simulink model "IOT_Charger"  (R2024b)
settings: Solver=ode23tb  StartTime=0.0  StopTime=1  RelTol=1e-3  EnableMultiTasking=on
PreLoadFcn:
  | % Data of Solar Panel
  | %5000[W]/130[W]
  | % Total power generated by solar panel reaches 5[KW].
  | % each solar panel generates power 130[kW].
  | V = [0    40 80 120 160 180 200 217 240 260 280];
  | I = 5000/130*[0.68 0.675 0.67 0.665 0.660 0.655 0.640 0.6 0.48 0.28 0];
  | 
  | %subplot(211);plot(V,I);xlabel('Voltage[V]');ylabel('Current[a]')
  | %subplot(212);plot(V.*I);title('Power[W]')
  | 
  | % Sample Time[s]
  | Ts =5e-6;
  | 
  | 
  | %MPPT + PV Control
  | % PI control pamameter of Voltage control(Outer loop)
  | Kp_V = 50e-3;
  | Ki_V = 10;
  | 
  | % PI Control pamameter of Current control(Inner loop)
  | Kp_I = 25e-3;
  | Ki_I = 10;
  | 
  | % Utility Interconnection Control
  | % PI Control pamameter of Voltage control(Outer loop)
  | Kp_V2 = 0.01;
  | Ki_V2 = 25;
  | 
  | % PI control pamameter of Current control(Inner loop)
  | Kp_I2 = 0.01;
  | Ki_I2 = 25;
  | 
  | 
  | % Difference of voltege using in MPPT
  | dV = 0.5;
  | 
  | % Battery Control
  | % PI Control pamameter of Voltage control(Outer loop)
  | Kp_VB = 0.4;
  | Ki_VB = 2;
  | 
  | % PI control pamameter of Current control(Inner loop)
  | Kp_IB = 0.1;
  | Ki_IB = 0.5;
undefined symbols (not defined in the file): Ion, Lithium, sigbuilder_block
libraries: spsBreakerLib x120, spsSeriesRLCBranchLib x72, spsBatteryLib x43, spsIdealSwitchLib x29, spsVoltageMeasurementLib x25, spsMosfetLib x19, slpidlib x17, spsSeriesRLCLoadLib x12, spsPWMGeneratorDCDCLib x11, spsCurrentMeasurementLib x10, spsDiodeLib x6, spsPWMGenerator2LevelLib x5
(part 1 of 6)
Description:
  | Copyright 2008-2017 The MathWorks, Inc.
settings Model: SimulationMode=accelerator  Creator=MathWorks  LastModifiedBy=Jatay
settings SolverCC: ZeroCrossControl=DisableAll  ZeroCrossAlgorithm=Adaptive  AlgebraicLoopSolver=TrustRegion
settings DataIOCC: LimitDataPoints=on  SaveFormat=Array  SignalLoggingSaveFormat=ModelDataLogs  ReturnWorkspaceOutputs=off
settings OptimizationCC: ExpressionDepthLimit=2147483647  LifeSpan=inf
settings DebuggingCC: UnderspecifiedInitializationDetection=Classic  MergeDetectMultiDrivingBlocksExec=none  SolverPrmCheckMsg=warning  FcnCallInpInsideContextMsg=warning  UnconnectedInputMsg=warning  UnconnectedOutputMsg=warning  UnconnectedLineMsg=warning  AllowSymbolicDim=off  StateNameClashWarn=warning  SFUnexpectedBacktrackingDiag=warning  SFNoUnconditionalDefaultTransitionDiag=warning  SFExecutionAtInitializationDiag=none  ArithmeticOperatorsInVariantConditions=warning
settings HardwareCC: ProdBitPerPointer=32  ProdBitPerSizeT=32  ProdBitPerPtrDiffT=32  ProdLargestAtomicFloat=None  ProdIntDivRoundTo=Undefined  ProdEndianess=Unspecified  ProdWordSize=32  ProdHWDeviceType=32-bit Generic
settings ModelReferenceCC: EnableRefExpFcnMdlSchedulingChecks=on  PropagateSignalLabelsOutOfModel=off
settings SFSimCC: SimUseLocalCustomCode=off  SimParseCustomCode=off  CustomCodeUndefinedFunction=UseInterfaceOnly
settings RTWCC: RTWUseLocalCustomCode=off  GPUComputeCapability=3.5
settings CodeAppCC: StateflowObjectComments=on
settings GRTTargetCC: TargetLangStandard=C89/C90 (ANSI)  CombineOutputUpdateFcns=off  GRTInterface=on
settings ConfigComp: CovMetricSettings=dw  CovSaveCumulativeToWorkspaceVar=on  CovSaveSingleToWorkspaceVar=on  CovExternalEMLEnable=off  CovSFcnEnable=off
settings SimscapeCC: SimscapeNormalizeSystem=off

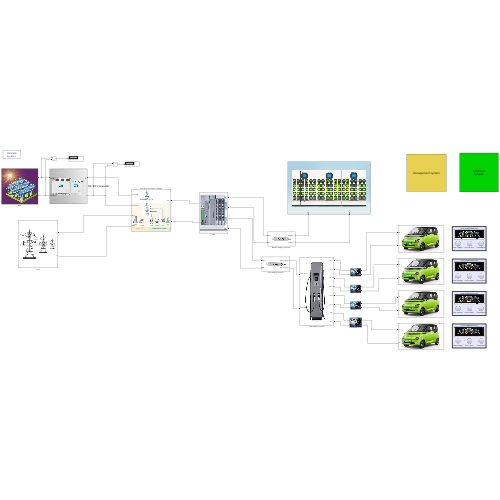
[thumbnail: Simulink's stored preview of the top-level diagram]
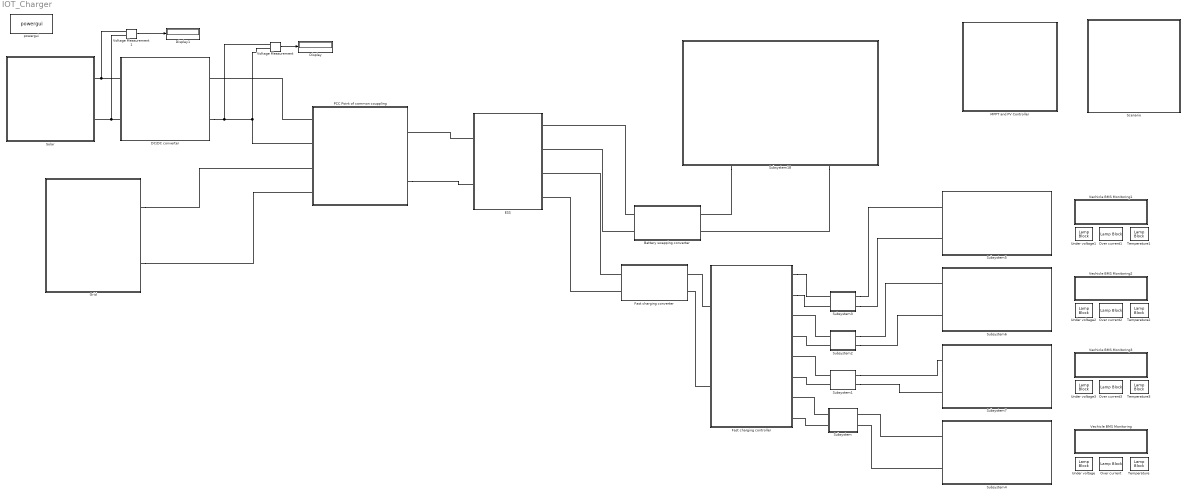
== system IOT_Charger ==
  Battery swapping converter : Subsystem
      mask Display: image('cc_converter.png');
  DC/DC converter : Subsystem
      mask Display: image('solar_controller.jpg');
  Display : Display
  Display1 : Display
  ESS : Subsystem
      mask Display: image('ess.jpeg');
  Fast charging controller : Subsystem
      mask Display: image('FC.jpeg');
  Fast charging converter : Subsystem
      mask Display: image('cc_converter.png');
  Grid : Subsystem
      mask Display: image('grid.png');
  MPPT and PV Controller : Subsystem
      mask Display: disp('Management system')
  Over current{,1..3} (4 alike) : LampBlock  LabelPosition=Hide
  PCC Point of common couppling : Subsystem
      mask Display: image('pcc.png');
  Scenario : Subsystem
      mask Display: disp('Additional\nScopes')
  Solar : Subsystem
      mask Display: image('Solar-Power-Plant-1024x536.jpg');
  Subsystem : Subsystem
      mask Display: image('plugin.jpeg');
  Subsystem1 : Subsystem
      mask Display: image('plugin.jpeg');
  Subsystem18 : Subsystem
      mask Display: image('swapping.webp');
  Subsystem2 : Subsystem
      mask Display: image('plugin.jpeg');
  Subsystem3 : Subsystem
      mask Display: image('plugin.jpeg');
  Subsystem4 : Subsystem
      mask Display: image('ev-1.jpeg');
  Subsystem5 : Subsystem
      mask Display: image('ev-1.jpeg');
  Subsystem6 : Subsystem
      mask Display: image('ev-1.jpeg');
  Subsystem7 : Subsystem
      mask Display: image('ev-1.jpeg');
  Temperature{,1..3} (4 alike) : LampBlock  LabelPosition=Hide
  Under voltage{,1..3} (4 alike) : LampBlock  LabelPosition=Hide
  Vechicle BMS Monitoring : Subsystem
      mask Display: image('Dash_board.jpeg');
  Vechicle BMS Monitoring1 : Subsystem
      mask Display: image('Dash_board.jpeg');
  Vechicle BMS Monitoring2 : Subsystem
      mask Display: image('Dash_board.jpeg');
  Vechicle BMS Monitoring3 : Subsystem
      mask Display: image('Dash_board.jpeg');
  Voltage Measurement : spsVoltageMeasurementLib/Voltage Measurement  PhasorSimulation=off  OutputType=Complex  PSBequivalent=0
  Voltage Measurement1 : spsVoltageMeasurementLib/Voltage Measurement  PhasorSimulation=off  OutputType=Complex  PSBequivalent=0
  powergui : spspowerguiLib/powergui  Priority=1  SimulationMode=Discrete  SampleTime=5e-6  frequency=60  Iterations=50  frequencyindice=0  Pbase=100e6  ErrMax=1e-4  UnitsV=kV  UnitsW=MW  buscounter=0  FunctionMessages=off  echomessages=off  EnableUseOfTLC=off  CurrentSourceSwitches=off  DisableSnubberDevices=off  DisableRonSwitches=off  DisableVfSwitches=off  DisplayEquations=off  AutomaticDiscreteSolvers=off  SolverType=Tustin  Interpol=off  ExternalGateDelay=off  methode=off  Ts=0  x0status=blocks  SPID=off  SwTol=0  HookPort=off  NonlinearTolerance=1e-4  nMaxIteration=100  ContinueOnMaxIteration=off  RestoreLinks=warning  ResistiveCurrentMeasurement=off  Frange=[0:2:500]  Ylog=off  Xlog=on  ShowGrid=off  save=off  variable=ZData  structure=0  ZoomFFT=off  StartTime=0.0  cycles=1  DisplayStyle=1  fundamental=60  FreqAxis=off  MaxFrequency=1000  frequencyindicesteady=1  RmsSteady=1  display=off
  wires:
  Voltage Measurement/1 -> Display/1
  Voltage Measurement1/1 -> Display1/1
  connections:
  DC/DC converter/LConn2 -- Voltage Measurement1/LConn2 -- Solar/RConn2
  DC/DC converter/LConn1 -- Voltage Measurement1/LConn1 -- Solar/RConn1
  PCC Point of common couppling/RConn2 -- ESS/LConn2
  ESS/LConn1 -- PCC Point of common couppling/RConn1
  PCC Point of common couppling/LConn1 -- DC/DC converter/RConn1
  DC/DC converter/RConn2 -- Voltage Measurement/LConn1 -- Voltage Measurement/LConn2 -- PCC Point of common couppling/LConn2
  Grid/RConn1 -- PCC Point of common couppling/LConn3
  Grid/RConn2 -- PCC Point of common couppling/LConn4
  Battery swapping converter/LConn1 -- ESS/RConn1
  Battery swapping converter/LConn2 -- ESS/RConn2
  Fast charging converter/LConn1 -- ESS/RConn3
  Fast charging converter/LConn2 -- ESS/RConn4
  Subsystem18/LConn1 -- Battery swapping converter/RConn1
  Subsystem18/LConn2 -- Battery swapping converter/RConn2
  Fast charging controller/LConn1 -- Fast charging converter/RConn2
  Fast charging controller/LConn2 -- Fast charging converter/RConn1
  Subsystem/LConn1 -- Fast charging controller/RConn2
  Subsystem/LConn2 -- Fast charging controller/RConn1
  Subsystem1/LConn2 -- Fast charging controller/RConn3
  Subsystem1/LConn1 -- Fast charging controller/RConn4
  Subsystem2/LConn2 -- Fast charging controller/RConn5
  Subsystem2/LConn1 -- Fast charging controller/RConn6
  Fast charging controller/RConn7 -- Subsystem3/LConn2
  Fast charging controller/RConn8 -- Subsystem3/LConn1
  Subsystem4/LConn1 -- Subsystem/RConn1
  Subsystem4/LConn2 -- Subsystem/RConn2
  Subsystem3/RConn1 -- Subsystem5/LConn1
  Subsystem3/RConn2 -- Subsystem5/LConn2
  Subsystem2/RConn1 -- Subsystem6/LConn1
  Subsystem2/RConn2 -- Subsystem6/LConn2
  Subsystem1/RConn1 -- Subsystem7/LConn1
  Subsystem1/RConn2 -- Subsystem7/LConn2

== system IOT_Charger/Battery swapping converter ==
  Current Measurement : spsCurrentMeasurementLib/Current Measurement  PhasorSimulation=off  OutputType=Complex  PSBequivalent=0
  Current Measurement1 : spsCurrentMeasurementLib/Current Measurement  PhasorSimulation=off  OutputType=Complex  PSBequivalent=0
  Current Measurement2 : spsCurrentMeasurementLib/Current Measurement  PhasorSimulation=off  OutputType=Complex  PSBequivalent=0
  Diode : spsDiodeLib/Diode  Ron=0.001  Lon=0  Vf=0.8  IC=0  UseSnubber=0  Rs=500  Cs=250e-9  Measurements=off
  Mosfet : spsMosfetLib/Mosfet  Ron=0.1  Lon=0  Rd=0.01  Vfd=0  IC=0  Rs=1e5  Cs=inf  Measurements=off
  Product : Product
  Pulse Generator : DiscretePulseGenerator  PulseType=Time based  Period=10  PulseWidth=5
  Scope2 : Scope  NumInputPorts=3
  Scope3 : Scope
  Scope4 : Scope
  Series RLC Branch : spsSeriesRLCBranchLib/Series RLC Branch  LConnTagsString=__new0  RConnTagsString=__new0  BranchType=L  Resistance=1  Inductance=1e-3  SetiL0=off  InitialCurrent=0  Capacitance=1e-6  Setx0=off  InitialVoltage=0  Measurements=None
  Series RLC Branch2 : spsSeriesRLCBranchLib/Series RLC Branch  LConnTagsString=__new0  RConnTagsString=__new0  BranchType=C  Resistance=1  Inductance=1e-3  SetiL0=off  InitialCurrent=0  Capacitance=1e-6  Setx0=off  InitialVoltage=0  Measurements=None
  Voltage Measurement : spsVoltageMeasurementLib/Voltage Measurement  PhasorSimulation=off  OutputType=Complex  PSBequivalent=0
  BB + : PMIOPort  Side=Left
  BB - : PMIOPort  Port=2  Side=Left
  Swapping + : PMIOPort  Port=3  Side=Right
  swapping - : PMIOPort  Port=4  Side=Right
  wires:
  Current Measurement/1 -> Scope2/1
  Voltage Measurement/1 -> Scope4/1, Product/1
  Current Measurement1/1 -> Scope2/3, Product/2
  Product/1 -> Scope3/1
  Current Measurement2/1 -> Scope2/2
  Pulse Generator/1 -> Mosfet/1
  connections:
  Series RLC Branch2/RConn1 -- BB -/RConn1 -- Series RLC Branch/RConn1 -- swapping -/RConn1 -- Voltage Measurement/LConn2
  Diode/LConn1 -- Current Measurement1/LConn1 -- Series RLC Branch2/LConn1
  BB +/RConn1 -- Current Measurement/LConn1
  Current Measurement1/RConn1 -- Swapping +/RConn1 -- Voltage Measurement/LConn1
  Mosfet/RConn1 -- Diode/RConn1 -- Current Measurement2/LConn1
  Current Measurement/RConn1 -- Mosfet/LConn1
  Current Measurement2/RConn1 -- Series RLC Branch/LConn1

== system IOT_Charger/DC//DC converter ==
  DC - DC Converter : Subsystem
  DC bus : Subsystem
  Display : Display
  Voltage Measurement : spsVoltageMeasurementLib/Voltage Measurement  PhasorSimulation=off  OutputType=Complex  PSBequivalent=0
  Voltage Measurement2 : spsVoltageMeasurementLib/Voltage Measurement  PhasorSimulation=off  OutputType=Complex  PSBequivalent=0
  solar + : PMIOPort  Side=Left
  solar - : PMIOPort  Port=2  Side=Left
  + : PMIOPort  Port=3  Side=Right
  - : PMIOPort  Port=4  Side=Right
  tag scope: solar_controller=global
  wires:
  Voltage Measurement2/1 -> [solar_controller]
  Voltage Measurement/1 -> Display/1
  connections:
  DC - DC Converter/RConn1 -- DC bus/LConn1
  solar +/RConn1 -- DC - DC Converter/LConn1 -- Voltage Measurement2/LConn1
  DC - DC Converter/LConn2 -- Voltage Measurement2/LConn2 -- solar -/RConn1
  DC - DC Converter/RConn2 -- DC bus/LConn2
  -/RConn1 -- DC bus/RConn2 -- Voltage Measurement/LConn2
  Voltage Measurement/LConn1 -- DC bus/RConn1 -- +/RConn1

== system IOT_Charger/ESS ==
  Battery : spsBatteryLib/Battery  BatType=Lithium-Ion  NomV=400  NomQ=40  SOC=80  Batt_Tr=30/10  PresetModel=on  MaxQ=40  MinV=300  FullV=465.5949  Dis_rate=17.3913  R=0.1  Normal_OP=36.1739  expZone="[432.1543      1.965217]"
  Battery Status : Scope  NumInputPorts=4
  Bus Selector : BusSelector  OutputSignals=SOC (%),Current (A),Voltage (V)
  Product1 : Product  RndMeth=Zero
  + : PMIOPort  Side=Left
  - : PMIOPort  Port=2  Side=Left
  BS + : PMIOPort  Port=3  Side=Right
  BS - : PMIOPort  Port=4  Side=Right
  FC + : PMIOPort  Port=5  Side=Right
  FC - : PMIOPort  Port=6  Side=Right
  tag scope: Power_Battery=global
  wires:
  Product1/1 -> [Power_Battery], Battery Status/4  "Power_Battery[W]"
  Battery/1 -> Bus Selector/1
  Bus Selector/3 -> Product1/2, Battery Status/3  "<Voltage (V)>"
  Bus Selector/2 -> Product1/1, Battery Status/2  "<Current (A)>"
  Bus Selector/1 -> Battery Status/1  "<SOC (%)>"
  connections:
  Battery/LConn2 -- -/RConn1 -- FC -/RConn1 -- BS -/RConn1
  Battery/LConn1 -- +/RConn1 -- FC +/RConn1 -- BS +/RConn1

== system IOT_Charger/Fast charging controller ==
  note: Solar
  Fast charging Switching controller : Subsystem
  Ideal Switch{,1..3} (4 alike) : spsIdealSwitchLib/Ideal Switch  Ron=0.001  Lon=0  IC=0  Rs=1e5  Cs=inf  Measurements=off
  solar panel - : PMIOPort  Side=Left
  solar panel + : PMIOPort  Port=2  Side=Left
  DC + : PMIOPort  Port=3  Side=Right
  DC - : PMIOPort  Port=4  Side=Right
  DC +1 : PMIOPort  Port=5  Side=Right
  DC +2 : PMIOPort  Port=6  Side=Right
  DC +3 : PMIOPort  Port=7  Side=Right
  DC +4 : PMIOPort  Port=8  Side=Right
  DC +5 : PMIOPort  Port=9  Side=Right
  DC +6 : PMIOPort  Port=10  Side=Right
  wires:
  [gg1] -> Ideal Switch3/1
  [gg2] -> Ideal Switch2/1
  [gg3] -> Ideal Switch1/1
  [gg4] -> Ideal Switch/1
  connections:
  Ideal Switch3/LConn1 -- Ideal Switch2/LConn1 -- Ideal Switch1/LConn1 -- Ideal Switch/LConn1 -- solar panel +/RConn1
  solar panel -/RConn1 -- DC +5/RConn1 -- DC +4/RConn1 -- DC +2/RConn1 -- DC -/RConn1
  Ideal Switch3/RConn1 -- DC +/RConn1
  Ideal Switch2/RConn1 -- DC +1/RConn1
  Ideal Switch1/RConn1 -- DC +3/RConn1
  Ideal Switch/RConn1 -- DC +6/RConn1

== system IOT_Charger/Fast charging converter ==
  Current Measurement : spsCurrentMeasurementLib/Current Measurement  PhasorSimulation=off  OutputType=Complex  PSBequivalent=0
  Current Measurement1 : spsCurrentMeasurementLib/Current Measurement  PhasorSimulation=off  OutputType=Complex  PSBequivalent=0
  Current Measurement2 : spsCurrentMeasurementLib/Current Measurement  PhasorSimulation=off  OutputType=Complex  PSBequivalent=0
  Diode : spsDiodeLib/Diode  Ron=0.001  Lon=0  Vf=0.8  IC=0  UseSnubber=0  Rs=500  Cs=250e-9  Measurements=off
  Mosfet : spsMosfetLib/Mosfet  Ron=0.1  Lon=0  Rd=0.01  Vfd=0  IC=0  Rs=1e5  Cs=inf  Measurements=off
  Product : Product
  Pulse Generator : DiscretePulseGenerator  PulseType=Time based  Period=10  PulseWidth=5
  Scope2 : Scope  NumInputPorts=3
  Scope3 : Scope
  Scope4 : Scope
  Series RLC Branch : spsSeriesRLCBranchLib/Series RLC Branch  LConnTagsString=__new0  RConnTagsString=__new0  BranchType=L  Resistance=1  Inductance=1e-3  SetiL0=off  InitialCurrent=0  Capacitance=1e-6  Setx0=off  InitialVoltage=0  Measurements=None
  Series RLC Branch2 : spsSeriesRLCBranchLib/Series RLC Branch  LConnTagsString=__new0  RConnTagsString=__new0  BranchType=C  Resistance=1  Inductance=1e-3  SetiL0=off  InitialCurrent=0  Capacitance=1e-6  Setx0=off  InitialVoltage=0  Measurements=None
  Voltage Measurement : spsVoltageMeasurementLib/Voltage Measurement  PhasorSimulation=off  OutputType=Complex  PSBequivalent=0
  BB + : PMIOPort  Side=Left
  BB - : PMIOPort  Port=2  Side=Left
  Fast charging + : PMIOPort  Port=3  Side=Right
  Fast charging - : PMIOPort  Port=4  Side=Right
  tag scope: FS=global
  wires:
  Current Measurement/1 -> Scope2/1
  Voltage Measurement/1 -> [FS], Scope4/1, Product/1
  Current Measurement1/1 -> Scope2/3, Product/2
  Product/1 -> Scope3/1
  Current Measurement2/1 -> Scope2/2
  Pulse Generator/1 -> Mosfet/1
  connections:
  Voltage Measurement/LConn2 -- Fast charging -/RConn1 -- Series RLC Branch2/RConn1 -- Series RLC Branch/RConn1 -- BB -/RConn1
  Diode/LConn1 -- Current Measurement1/LConn1 -- Series RLC Branch2/LConn1
  BB +/RConn1 -- Current Measurement/LConn1
  Current Measurement1/RConn1 -- Voltage Measurement/LConn1 -- Fast charging +/RConn1
  Mosfet/RConn1 -- Diode/RConn1 -- Current Measurement2/LConn1
  Current Measurement/RConn1 -- Mosfet/LConn1
  Current Measurement2/RConn1 -- Series RLC Branch/LConn1

== system IOT_Charger/Grid ==
  Display : Display
  Grid : spsThreePhaseSourceLib/Three-Phase Source  InternalConnection=Yg  VoltagePhases=off  Voltage=380  PhaseAngle=0  Voltage_phases=[25e3 25e3 25e3]/sqrt(3)  PhaseAngles_phases=[0 -120 +120]  Frequency=50  NonIdealSource=on  SpecifyImpedance=on  Resistance=0.8929  Inductance=16.58e-3  ShortCircuitLevel=100e6  BaseVoltage=380  XRratio=7  BusType=swing  Pref=10e3  Qref=0  Prefabc=[10e3, 10e3, 10e3]  Qrefabc=[0, 0, 0]  Qmin=-inf  Qmax=inf
  LOAD1 : spsThreePhaseSeriesRLCLoadLib/Three-Phase Series RLC Load  LConnTagsString=A|B|C  Configuration=Y (grounded)  NominalVoltage=380  Vabc=[1e3 1e3 1e3]  Vabcp=[1e3 1e3 1e3]  NominalFrequency=50  UnbalancedPower=off  ActivePower=1e3  InductivePower=0  CapacitivePower=0  Pabc=[10e3 9e3 11e3]  QLabc=[100 90 110]  QCabc=[100 90 110]  Pabcp=[10e3 9e3 11e3]  QLabcp=[100 90 110]  QCabcp=[100 90 110]  Measurements=None  LoadType=constant Z
  Measurement : spsThreePhaseVIMeasurementLib/Three-Phase V-I Measurement  VoltageMeasurement=phase-to-phase  SetLabelV=on  LabelV=Vabc_grid  Vpu=off  VpuLL=off  CurrentMeasurement=yes  SetLabelI=on  LabelI=Iabc_grid  Ipu=off  Pbase=100e6  Vbase=500e3  OutputType=Complex  PhasorSimulation=off  PSBequivalent=0
  Mux : Mux  Inputs=2
  Repeating Sequence Stair : simulink/Sources/Repeating Sequence Stair  OutValues=[0 0 1 1 0].'  tsamp=0.1  OutMin=[]  OutMax=[]  OutDataTypeStr=double  OutputDataTypeScalingMode=double  OutDataType=fixdt(0,8)  ConRadixGroup=Best Precision: Vector-wise  OutScaling=2^-12
  Scope : Scope
  Scope1 : Scope
  Scope2 : Scope  NumInputPorts=2
  V2G & G2V results : Scope  NumInputPorts=3
  Voltage Measurement : spsVoltageMeasurementLib/Voltage Measurement  PhasorSimulation=off  OutputType=Complex  PSBequivalent=0
  Wall charger Connection Box : Subsystem
  + : PMIOPort  Side=Right
  +1 : PMIOPort  Port=2  Side=Right
  tag scope: Control=global
  wires:
  [Control] -> Wall charger Connection Box/1(Control)
  Mux/1 -> V2G & G2V results/3
  [Vabc_grid] -> V2G & G2V results/1
  [Vabc_inv] -> V2G & G2V results/2
  Repeating Sequence Stair/1 -> [Control], Scope1/1
  [Vabc_inv] -> Mux/2
  [Iabc_out] -> Scope2/2
  [Iabc_inv] -> Scope/1
  [Vabc_out] -> Scope2/1
  Voltage Measurement/1 -> Display/1
  [Vabc_grid] -> Mux/1
  connections:
  Wall charger Connection Box/RConn2 -- Voltage Measurement/LConn2 -- +1/RConn1
  Grid/RConn1 -- Measurement/LConn1
  Grid/RConn3 -- Measurement/LConn3
  Wall charger Connection Box/RConn1 -- Voltage Measurement/LConn1 -- +/RConn1
  Grid/RConn2 -- Measurement/LConn2
  LOAD1/LConn3 -- Measurement/RConn3 -- Wall charger Connection Box/LConn3
  Measurement/RConn2 -- LOAD1/LConn2 -- Wall charger Connection Box/LConn2
  Measurement/RConn1 -- LOAD1/LConn1 -- Wall charger Connection Box/LConn1

== system IOT_Charger/MPPT and PV Controller ==
  Battery controller : Subsystem
  Inverter controller : Subsystem
  MMPT Controller : Subsystem
  Solar controller : Subsystem
  Swapping battery controller : Subsystem

== system IOT_Charger/PCC Point of common couppling ==
  note: ESS
  note: Grid
  note: Solar
  Display : Display
  Display1 : Display
  Display2 : Display
  Voltage Measurement : spsVoltageMeasurementLib/Voltage Measurement  PhasorSimulation=off  OutputType=Complex  PSBequivalent=0
  Voltage Measurement1 : spsVoltageMeasurementLib/Voltage Measurement  PhasorSimulation=off  OutputType=Complex  PSBequivalent=0
  Voltage Measurement2 : spsVoltageMeasurementLib/Voltage Measurement  PhasorSimulation=off  OutputType=Complex  PSBequivalent=0
  DC + : PMIOPort  Side=Right
  solar panel + : PMIOPort  Port=2  Side=Left
  solar panel - : PMIOPort  Port=3  Side=Left
  DC - : PMIOPort  Port=4  Side=Right
  Grid + : PMIOPort  Port=5  Side=Left
  Grid - : PMIOPort  Port=6  Side=Left
  wires:
  Voltage Measurement/1 -> Display/1
  Voltage Measurement1/1 -> Display1/1
  Voltage Measurement2/1 -> Display2/1
  connections:
  DC +/RConn1 -- Voltage Measurement2/LConn1 -- Voltage Measurement1/LConn1 -- Grid +/RConn1 -- Voltage Measurement/LConn1 -- solar panel +/RConn1
  solar panel -/RConn1 -- Voltage Measurement/LConn2 -- Grid -/RConn1 -- Voltage Measurement1/LConn2 -- Voltage Measurement2/LConn2 -- DC -/RConn1

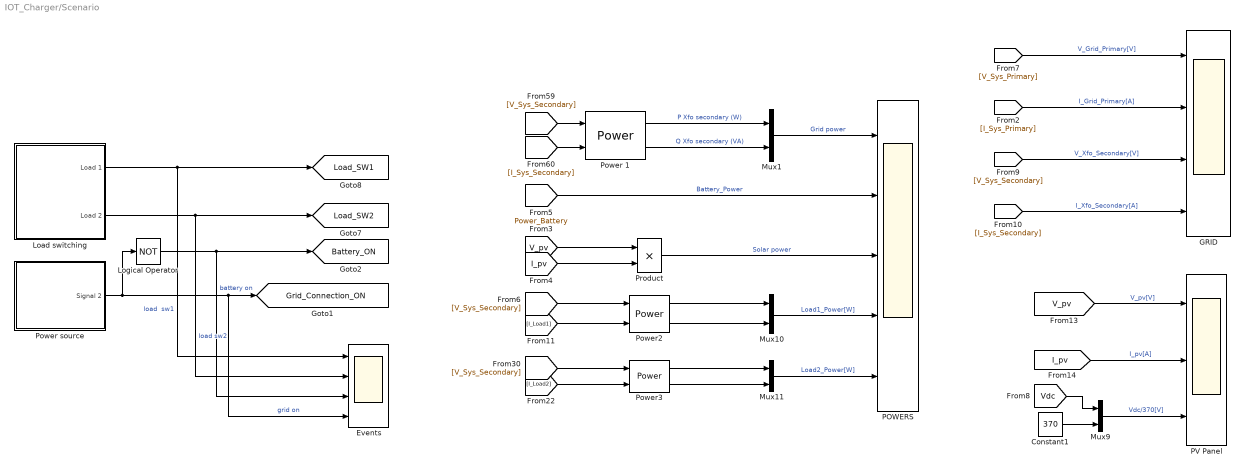
== system IOT_Charger/Scenario ==
  Constant1 : Constant  Value=370
  Events : Scope  NumInputPorts=4
  GRID : Scope  NumInputPorts=4
  Load switching : Subsystem  Tag=STV Subsys  LoadFcn=sigbuilder_block('load');  StartFcn=sigbuilder_block('start');  StopFcn=sigbuilder_block('stop');  ClipboardFcn=sigbuilder_block('clipboard');  mask(Sigbuilder block){tuvar=[0:10]}
      mask help: Simulink:masks:SigbuilderBlock_MD
      mask init:
      | if ~strcmp(get_param(bdroot(gcbh),'SimulationStatus'),'stopped') tuvar = sigbuilder_block('maskInit'); end
      settings: CopyFcn=sigbuilder_block('copy');  DeleteFcn=sigbuilder_block('delete');  ModelCloseFcn=sigbuilder_block('modelClose');  PreSaveFcn=sigbuilder_block('preSave');  PauseFcn=sigbuilder_block('pause');  ContinueFcn=sigbuilder_block('continue');  NameChangeFcn=sigbuilder_block('namechange');  OpenFcn=sigbuilder_block('open',[57 105.75 1180.5 663.75 ]);  CloseFcn=sigbuilder_block('close');
      mask Display: plot(0, 0, 100, 100,[2, 2, 32, 32, 2], [68, 8, 8, 68, 68],[32, 2], [38, 38], [32, 19, 2],[53, 60, 44], [32, 17, 17, 2],[16, 16, 31, 31]);txt = getActiveGroup(gcbh);text(2, 100, txt,'verticalAlignment', 'top');
  Logical Operator : Logic  Operator=NOT  AllPortsSameDT=off  OutDataTypeStr=boolean
  Mux{1,9..11} (4 alike) : Mux  Inputs=2
  POWERS : Scope  NumInputPorts=5
  PV Panel : Scope  NumInputPorts=3
  Power 1 : spsPowerLib/Power  Freq=60  Vinit=[1, 0]  Iinit=[1, 0]  Ts=0
  Power source : Subsystem  Tag=STV Subsys  LoadFcn=sigbuilder_block('load');  StartFcn=sigbuilder_block('start');  StopFcn=sigbuilder_block('stop');  ClipboardFcn=sigbuilder_block('clipboard');  mask(Sigbuilder block){tuvar=[0:10]}
      mask help: Simulink:masks:SigbuilderBlock_MD
      mask init:
      | if ~strcmp(get_param(bdroot(gcbh),'SimulationStatus'),'stopped') tuvar = sigbuilder_block('maskInit'); end
      settings: CopyFcn=sigbuilder_block('copy');  DeleteFcn=sigbuilder_block('delete');  ModelCloseFcn=sigbuilder_block('modelClose');  PreSaveFcn=sigbuilder_block('preSave');  PauseFcn=sigbuilder_block('pause');  ContinueFcn=sigbuilder_block('continue');  NameChangeFcn=sigbuilder_block('namechange');  OpenFcn=sigbuilder_block('open',[436.966 199.241 549.931 400.345 ]);  CloseFcn=sigbuilder_block('close');
      mask Display: plot(0, 0, 100, 100,[2, 2, 32, 32, 2], [68, 8, 8, 68, 68],[32, 2], [38, 38], [32, 19, 2],[53, 60, 44], [32, 17, 17, 2],[16, 16, 31, 31]);txt = getActiveGroup(gcbh);text(2, 100, txt,'verticalAlignment', 'top');
  Power2 : spsPowerLib/Power  Freq=60  Vinit=[1, 0]  Iinit=[1, 0]  Ts=0
  Power3 : spsPowerLib/Power  Freq=60  Vinit=[1, 0]  Iinit=[1, 0]  Ts=0
  Product : Product  RndMeth=Zero
  tag scope: Battery_ON=global, Grid_Connection_ON=global, Load_SW1=global, Load_SW2=global
  wires:
  Load switching/2(Load 2) -> [Load_SW2], Events/2  "load sw2"
  Logical Operator/1 -> Events/3, [Battery_ON]  "battery on"
  Power source/1(Signal 2) -> Events/4, [Grid_Connection_ON], Logical Operator/1  "grid on"
  Load switching/1(Load 1) -> [Load_SW1], Events/1  "load  sw1"
  [Vdc] -> Mux9/1
  Constant1/1 -> Mux9/2
  Mux9/1 -> PV Panel/3  "Vdc/370[V]"
  [V_Sys_Primary] -> GRID/1  "V_Grid_Primary[V]"
  [I_Sys_Primary] -> GRID/2  "I_Grid_Primary[A]"
  [V_Sys_Secondary] -> GRID/3  "V_Xfo_Secondary[V]"
  [I_Sys_Secondary] -> GRID/4  "I_Xfo_Secondary[A]"
  [V_pv] -> PV Panel/1  "V_pv[V]"
  [I_pv] -> PV Panel/2  "I_pv[A]"
  [V_pv] -> Product/1
  [I_pv] -> Product/2
  Product/1 -> POWERS/3  "Solar power"
  [Power_Battery] -> POWERS/2  "Battery_Power"
  [V_Sys_Secondary] -> Power 1/1
  [I_Sys_Secondary] -> Power 1/2
  [V_Sys_Secondary] -> Power2/1
  [I_Load1] -> Power2/2
  Mux10/1 -> POWERS/4  "Load1_Power[W]"
  [V_Sys_Secondary] -> Power3/1
  [I_Load2] -> Power3/2
  Mux11/1 -> POWERS/5  "Load2_Power[W]"
  Power2/1 -> Mux10/1
  Power2/2 -> Mux10/2
  Power3/1 -> Mux11/1
  Power3/2 -> Mux11/2
  Mux1/1 -> POWERS/1  "Grid power"
  Power 1/1 -> Mux1/1  "P Xfo secondary (W)"
  Power 1/2 -> Mux1/2  "Q Xfo secondary (VA)"

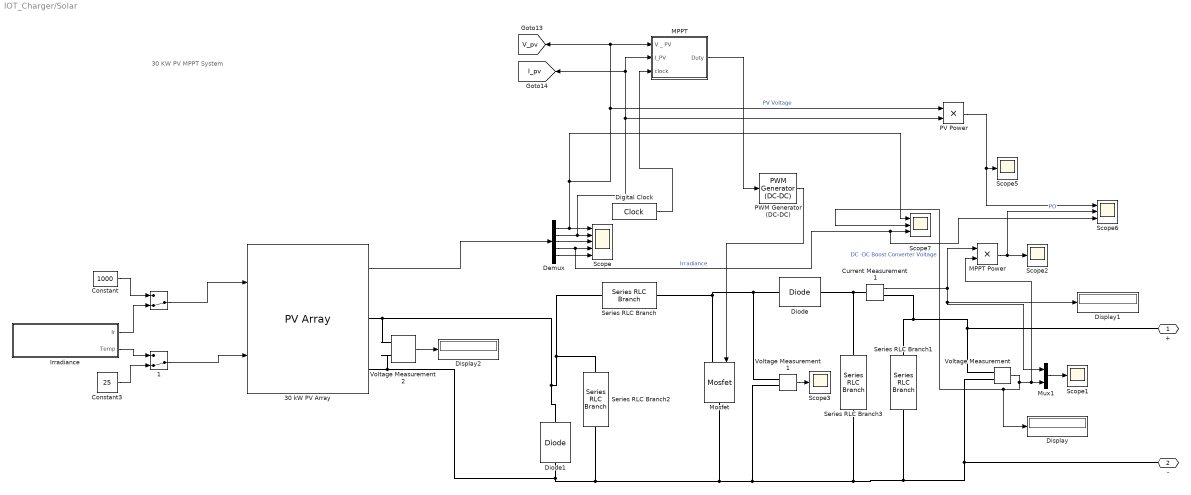
== system IOT_Charger/Solar ==
  note: 30 KW PV MPPT System
  "      " : ManualSwitch  CurrentSetting=0
  "      1" : ManualSwitch  CurrentSetting=0
  30 kW PV Array : spsPVArrayLib/PV Array  Npar=15  Nser=10  PlotType=array @ 1000 W/m2 & specified temperatures  S_vec="[ 1000  500  100 ]"  Temp_C_vec="[ 45 25  ]"  ModuleName=User-defined  PlotWhenSelected=off  Pm=213.15  Ncell=60  Voc=48  Isc=7.84  Vm=29  Im=7.35  beta_Voc_pc=-0.36099  alpha_Isc_pc=0.102  beta_Voc=-0.17328  alpha_Isc=0.0079968  IL=8.2285  I0=2.9956e-10  nI=1.2955  Rsh=7353.5939  Rs=2.0228  RobustModel=off  RobustCellTemperature=25  BAL=on  Tc=1e-6  Tfilter=5e-5
  Constant : Constant  Value=1000
  Constant3 : Constant  Value=25
  Current Measurement1 : spsCurrentMeasurementLib/Current Measurement  PhasorSimulation=off  OutputType=Complex  PSBequivalent=0
  Demux : Demux  Outputs=5
  Digital Clock : DigitalClock  SampleTime=0.001
  Diode : spsDiodeLib/Diode  Ron=0.5  Lon=0  Vf=0.7  IC=0  UseSnubber=0  Rs=1e5  Cs=250e-9  Measurements=off
  Diode1 : spsDiodeLib/Diode  Ron=0.5  Lon=0  Vf=0.7  IC=0  UseSnubber=0  Rs=1e5  Cs=250e-9  Measurements=off
  Display : Display
  Display1 : Display
  Display2 : Display
  "Irradiance " : Subsystem  Tag=STV Subsys  LoadFcn=sigbuilder_block('load');  StartFcn=sigbuilder_block('start');  StopFcn=sigbuilder_block('stop');  ClipboardFcn=sigbuilder_block('clipboard');  mask(Sigbuilder block){tuvar=[0:10]}
      mask help: Sigbuilder GUI
      mask init:
      | if ~strcmp(get_param(bdroot(gcbh),'SimulationStatus'),'stopped') tuvar = sigbuilder_block('maskInit'); end
      settings: CopyFcn=sigbuilder_block('copy');  DeleteFcn=sigbuilder_block('delete');  ModelCloseFcn=sigbuilder_block('modelClose');  PreSaveFcn=sigbuilder_block('preSave');  PauseFcn=sigbuilder_block('pause')  ContinueFcn=sigbuilder_block('continue')  NameChangeFcn=sigbuilder_block('namechange');  OpenFcn=sigbuilder_block('open',[5.4 30 1141.2 507.6 ]);  CloseFcn=sigbuilder_block('close');
      mask Display: plot(0, 0, 100, 100,[2, 2, 32, 32, 2], [68, 8, 8, 68, 68],[32, 2], [38, 38], [32, 19, 2],[53, 60, 44], [32, 17, 17, 2],[16, 16, 31, 31]);txt = getActiveGroup(gcbh);text(2, 100, txt,'verticalAlignment', 'top');
  MPPT : Subsystem
  MPPT Power : Product
  Mosfet : spsMosfetLib/Mosfet  Ron=0.1  Lon=0  Rd=0.01  Vfd=0.7  IC=0  Rs=1e5  Cs=inf  Measurements=off
  Mux1 : Mux  Inputs=2
  PV Power : Product
  PWM Generator (DC-DC) : spsPWMGeneratorDCDCLib/PWM Generator (DC-DC)  Fsw=1500  Ts=0
  Scope : Scope  NumInputPorts=5
  Scope{1..3,5} (4 alike) : Scope
  Scope6 : Scope  NumInputPorts=3
  Scope7 : Scope  NumInputPorts=3
  Series RLC Branch : spsSeriesRLCBranchLib/Series RLC Branch  LConnTagsString=__new0  RConnTagsString=__new0  BranchType=L  Resistance=0.001  Inductance=0.4e-1  SetiL0=off  InitialCurrent=0  Capacitance=1e-6  Setx0=off  InitialVoltage=0  Measurements=None
  Series RLC Branch1 : spsSeriesRLCBranchLib/Series RLC Branch  LConnTagsString=__new0  RConnTagsString=__new0  BranchType=R  Resistance=11  Inductance=0.1  SetiL0=off  InitialCurrent=0  Capacitance=100e-6  Setx0=off  InitialVoltage=0  Measurements=None
  Series RLC Branch2 : spsSeriesRLCBranchLib/Series RLC Branch  LConnTagsString=__new0  RConnTagsString=__new0  BranchType=C  Resistance=6  Inductance=0.1  SetiL0=off  InitialCurrent=0  Capacitance=700e-5  Setx0=off  InitialVoltage=0  Measurements=None
  Series RLC Branch3 : spsSeriesRLCBranchLib/Series RLC Branch  LConnTagsString=__new0  RConnTagsString=__new0  BranchType=C  Resistance=6  Inductance=0.1  SetiL0=off  InitialCurrent=0  Capacitance=1000e-5  Setx0=off  InitialVoltage=0  Measurements=None
  Voltage Measurement : spsVoltageMeasurementLib/Voltage Measurement  PhasorSimulation=off  OutputType=Complex  PSBequivalent=0
  Voltage Measurement1 : spsVoltageMeasurementLib/Voltage Measurement  PhasorSimulation=off  OutputType=Complex  PSBequivalent=0
  Voltage Measurement2 : spsVoltageMeasurementLib/Voltage Measurement  PhasorSimulation=off  OutputType=Complex  PSBequivalent=0
  + : PMIOPort  Side=Right
  - : PMIOPort  Port=2  Side=Right
  tag scope: I_pv=global, V_pv=global
  wires:
  Voltage Measurement/1 -> MPPT Power/2, Mux1/2, Display/1, Scope7/2  "DC -DC Boost Converter Voltage"
  PWM Generator (DC-DC)/1 -> Mosfet/1
  Demux/1 -> Scope7/1, PV Power/1, [V_pv], MPPT/1("V _ PV "), Scope/1  "PV Voltage"
  Mux1/1 -> Scope1/1
  MPPT Power/1 -> Scope6/2, Scope2/1  "PO"
  Demux/2 -> PV Power/2, [I_pv], MPPT/2(I_PV), Scope/2
  Current Measurement1/1 -> MPPT Power/1, Display1/1, Mux1/1
  Voltage Measurement1/1 -> Scope3/1
  Demux/3 -> Scope/3
  Demux/4 -> Scope6/3, Scope7/3, Scope/4  "Irradiance"
  Digital Clock/1 -> MPPT/3(clock)
  MPPT/1(Duty) -> PWM Generator (DC-DC)/1
  PV Power/1 -> Scope6/1, Scope5/1
  Demux/5 -> Scope/5
  "Irradiance "/2(Temp) -> "      1"/1
  Constant3/1 -> "      1"/2
  "Irradiance "/1(Ir) -> "      "/2
  Constant/1 -> "      "/1
  "      "/1 -> 30 kW PV Array/1
  "      1"/1 -> 30 kW PV Array/2
  30 kW PV Array/1 -> Demux/1
  Voltage Measurement2/1 -> Display2/1
  connections:
  Voltage Measurement/LConn2 -- Voltage Measurement2/LConn2 -- 30 kW PV Array/RConn2 -- Diode1/LConn1 -- Series RLC Branch2/RConn1 -- Mosfet/RConn1 -- Voltage Measurement1/LConn2 -- Series RLC Branch3/RConn1 -- Series RLC Branch1/RConn1 -- -/RConn1
  Current Measurement1/RConn1 -- Series RLC Branch1/LConn1 -- Voltage Measurement/LConn1 -- +/RConn1
  Diode/RConn1 -- Series RLC Branch3/LConn1 -- Current Measurement1/LConn1
  Voltage Measurement1/LConn1 -- Series RLC Branch/RConn1 -- Mosfet/LConn1 -- Diode/LConn1
  Series RLC Branch2/LConn1 -- Voltage Measurement2/LConn1 -- 30 kW PV Array/RConn1 -- Diode1/RConn1 -- Series RLC Branch/LConn1

== system IOT_Charger/Subsystem ==
  1 : spsMosfetLib/Mosfet  Ron=0.1  Lon=0  Rd=0.01  Vfd=0  IC=0  Rs=1e5  Cs=inf  Measurements=off
  2 : spsMosfetLib/Mosfet  Ron=0.1  Lon=0  Rd=0.01  Vfd=0  IC=0  Rs=1e5  Cs=inf  Measurements=off
  Constant : Constant
  Control : Subsystem
  Ideal Switch : spsIdealSwitchLib/Ideal Switch  Ron=0.001  Lon=0  IC=0  Rs=1e5  Cs=inf  Measurements=off
  Series RLC Branch : spsSeriesRLCBranchLib/Series RLC Branch  LConnTagsString=__new0  RConnTagsString=__new0  BranchType=RL  Resistance=0.05  Inductance=5.76e-3  SetiL0=off  InitialCurrent=0  Capacitance=1e-6  Setx0=off  InitialVoltage=0  Measurements=None
  Series RLC Branch1 : spsSeriesRLCBranchLib/Series RLC Branch  LConnTagsString=__new0  RConnTagsString=__new0  BranchType=R  Resistance=5  Inductance=5.76e-4  SetiL0=off  InitialCurrent=0  Capacitance=1e-6  Setx0=off  InitialVoltage=0  Measurements=None
  Series RLC Branch2 : spsSeriesRLCBranchLib/Series RLC Branch  LConnTagsString=__new0  RConnTagsString=__new0  BranchType=RC  Resistance=0.001  Inductance=5.76e-4  SetiL0=off  InitialCurrent=0  Capacitance=1000e-6  Setx0=off  InitialVoltage=0  Measurements=None
  bb - : PMIOPort  Side=Left
  bb + : PMIOPort  Port=2  Side=Left
  vv_1 + : PMIOPort  Port=3  Side=Right
  vv_2 - : PMIOPort  Port=4  Side=Right
  wires:
  [Mosfet_1] -> 1/1
  [Mosfet_2] -> 2/1
  Constant/1 -> Ideal Switch/1
  connections:
  Series RLC Branch2/LConn1 -- Series RLC Branch1/LConn1 -- Ideal Switch/RConn1 -- 1/LConn1
  2/RConn1 -- vv_2 -/RConn1 -- bb -/RConn1 -- Series RLC Branch1/RConn1 -- Series RLC Branch2/RConn1
  1/RConn1 -- 2/LConn1 -- Series RLC Branch/LConn1
  Series RLC Branch/RConn1 -- vv_1 +/RConn1
  bb +/RConn1 -- Ideal Switch/LConn1

== system IOT_Charger/Subsystem1 ==
  1 : spsMosfetLib/Mosfet  Ron=0.1  Lon=0  Rd=0.01  Vfd=0  IC=0  Rs=1e5  Cs=inf  Measurements=off
  2 : spsMosfetLib/Mosfet  Ron=0.1  Lon=0  Rd=0.01  Vfd=0  IC=0  Rs=1e5  Cs=inf  Measurements=off
  Constant : Constant
  Control : Subsystem
  Ideal Switch : spsIdealSwitchLib/Ideal Switch  Ron=0.001  Lon=0  IC=0  Rs=1e5  Cs=inf  Measurements=off
  Series RLC Branch : spsSeriesRLCBranchLib/Series RLC Branch  LConnTagsString=__new0  RConnTagsString=__new0  BranchType=RL  Resistance=0.05  Inductance=5.76e-3  SetiL0=off  InitialCurrent=0  Capacitance=1e-6  Setx0=off  InitialVoltage=0  Measurements=None
  Series RLC Branch1 : spsSeriesRLCBranchLib/Series RLC Branch  LConnTagsString=__new0  RConnTagsString=__new0  BranchType=R  Resistance=5  Inductance=5.76e-4  SetiL0=off  InitialCurrent=0  Capacitance=1e-6  Setx0=off  InitialVoltage=0  Measurements=None
  Series RLC Branch2 : spsSeriesRLCBranchLib/Series RLC Branch  LConnTagsString=__new0  RConnTagsString=__new0  BranchType=RC  Resistance=0.001  Inductance=5.76e-4  SetiL0=off  InitialCurrent=0  Capacitance=1000e-6  Setx0=off  InitialVoltage=0  Measurements=None
  bb - : PMIOPort  Side=Left
  bb + : PMIOPort  Port=2  Side=Left
  vv_1 + : PMIOPort  Port=3  Side=Right
  vv_2 - : PMIOPort  Port=4  Side=Right
  wires:
  [Mosfet_22] -> 1/1
  [Mosfet_222] -> 2/1
  Constant/1 -> Ideal Switch/1
  connections:
  Series RLC Branch2/LConn1 -- Series RLC Branch1/LConn1 -- Ideal Switch/RConn1 -- 1/LConn1
  bb -/RConn1 -- Series RLC Branch1/RConn1 -- Series RLC Branch2/RConn1 -- 2/RConn1 -- vv_2 -/RConn1
  1/RConn1 -- Series RLC Branch/LConn1 -- 2/LConn1
  Series RLC Branch/RConn1 -- vv_1 +/RConn1
  bb +/RConn1 -- Ideal Switch/LConn1

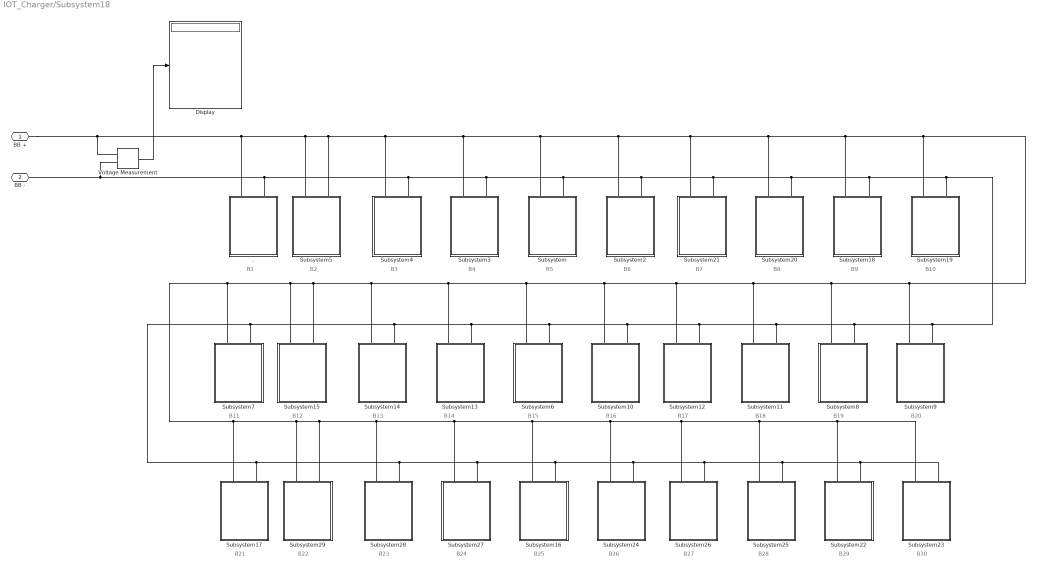
== system IOT_Charger/Subsystem18 ==
  note: B1
  note: B2
  note: B3
  note: B4
  note: B5
  note: B6
  note: B13
  note: B14
  note: B15
  note: B16
  note: B17
  note: B18
  note: B19
  note: B20
  note: B21
  note: B22
  note: B7
  note: B8
  note: B9
  note: B10
  note: B11
  note: B12
  note: B23
  note: B24
  note: B25
  note: B26
  note: B27
  note: B28
  note: B29
  note: B30
  . : Subsystem
  Display : Display
      settings: Decimation=2
  Subsystem : Subsystem
  Subsystem10 : Subsystem
  Subsystem11 : Subsystem
  Subsystem12 : Subsystem
  Subsystem13 : Subsystem
  Subsystem14 : Subsystem
  Subsystem15 : Subsystem
  Subsystem16 : Subsystem
  Subsystem17 : Subsystem
  Subsystem18 : Subsystem
  Subsystem19 : Subsystem
  Subsystem2 : Subsystem
  Subsystem20 : Subsystem
  Subsystem21 : Subsystem
  Subsystem22 : Subsystem
  Subsystem23 : Subsystem
  Subsystem24 : Subsystem
  Subsystem25 : Subsystem
  Subsystem26 : Subsystem
  Subsystem27 : Subsystem
  Subsystem28 : Subsystem
  Subsystem29 : Subsystem
  Subsystem3 : Subsystem
  Subsystem4 : Subsystem
  Subsystem5 : Subsystem
  Subsystem6 : Subsystem
  Subsystem7 : Subsystem
  Subsystem8 : Subsystem
  Subsystem9 : Subsystem
  Voltage Measurement : spsVoltageMeasurementLib/Voltage Measurement  PhasorSimulation=off  OutputType=Complex  PSBequivalent=0
  BB + : PMIOPort  Side=Left
  BB - : PMIOPort  Port=2  Side=Left
  wires:
  Voltage Measurement/1 -> Display/1
  connections:
  ./RConn2 -- Subsystem21/RConn2 -- Subsystem19/RConn2 -- Subsystem9/RConn2 -- Subsystem8/RConn2 -- Subsystem11/RConn2 -- Subsystem12/RConn2 -- Subsystem10/RConn2 -- Subsystem6/RConn2 -- Subsystem13/RConn2 -- Subsystem14/RConn2 -- Subsystem7/RConn2 -- Subsystem17/RConn2 -- Subsystem28/RConn2 -- Subsystem27/RConn2 -- Subsystem16/RConn2 -- Subsystem26/RConn2 -- Subsystem23/RConn2 -- Subsystem22/RConn2 -- Subsystem25/RConn2 -- Subsystem24/RConn2 -- Subsystem18/RConn2 -- Subsystem20/RConn2 -- Subsystem2/RConn2 -- Subsystem/RConn2 -- Subsystem3/RConn2 -- Subsystem4/RConn2 -- Voltage Measurement/LConn2 -- BB -/RConn1
  Subsystem10/RConn1 -- Subsystem7/RConn1 -- Subsystem17/RConn1 -- Subsystem29/RConn1 -- Subsystem29/RConn2 -- Subsystem28/RConn1 -- Subsystem27/RConn1 -- Subsystem16/RConn1 -- Subsystem26/RConn1 -- Subsystem25/RConn1 -- Subsystem22/RConn1 -- Subsystem23/RConn1 -- Subsystem24/RConn1 -- Subsystem15/RConn1 -- Subsystem15/RConn2 -- Subsystem14/RConn1 -- Subsystem13/RConn1 -- Subsystem6/RConn1 -- Subsystem12/RConn1 -- Subsystem11/RConn1 -- Subsystem8/RConn1 -- Subsystem20/RConn1 -- Voltage Measurement/LConn1 -- BB +/RConn1 -- ./RConn1 -- Subsystem5/RConn1 -- Subsystem5/RConn2 -- Subsystem4/RConn1 -- Subsystem3/RConn1 -- Subsystem/RConn1 -- Subsystem2/RConn1 -- Subsystem21/RConn1 -- Subsystem18/RConn1 -- Subsystem19/RConn1 -- Subsystem9/RConn1

== system IOT_Charger/Subsystem2 ==
  1 : spsMosfetLib/Mosfet  Ron=0.1  Lon=0  Rd=0.01  Vfd=0  IC=0  Rs=1e5  Cs=inf  Measurements=off
  2 : spsMosfetLib/Mosfet  Ron=0.1  Lon=0  Rd=0.01  Vfd=0  IC=0  Rs=1e5  Cs=inf  Measurements=off
  Constant : Constant
  Control : Subsystem
  Ideal Switch : spsIdealSwitchLib/Ideal Switch  Ron=0.001  Lon=0  IC=0  Rs=1e5  Cs=inf  Measurements=off
  Series RLC Branch : spsSeriesRLCBranchLib/Series RLC Branch  LConnTagsString=__new0  RConnTagsString=__new0  BranchType=RL  Resistance=0.05  Inductance=5.76e-3  SetiL0=off  InitialCurrent=0  Capacitance=1e-6  Setx0=off  InitialVoltage=0  Measurements=None
  Series RLC Branch1 : spsSeriesRLCBranchLib/Series RLC Branch  LConnTagsString=__new0  RConnTagsString=__new0  BranchType=R  Resistance=5  Inductance=5.76e-4  SetiL0=off  InitialCurrent=0  Capacitance=1e-6  Setx0=off  InitialVoltage=0  Measurements=None
  Series RLC Branch2 : spsSeriesRLCBranchLib/Series RLC Branch  LConnTagsString=__new0  RConnTagsString=__new0  BranchType=RC  Resistance=0.001  Inductance=5.76e-4  SetiL0=off  InitialCurrent=0  Capacitance=1000e-6  Setx0=off  InitialVoltage=0  Measurements=None
  bb - : PMIOPort  Side=Left
  bb + : PMIOPort  Port=2  Side=Left
  vv_1 + : PMIOPort  Port=3  Side=Right
  vv_2 - : PMIOPort  Port=4  Side=Right
  wires:
  [Mosfet_33] -> 1/1
  [Mosfet_333] -> 2/1
  Constant/1 -> Ideal Switch/1
  connections:
  Series RLC Branch2/LConn1 -- Series RLC Branch1/LConn1 -- Ideal Switch/RConn1 -- 1/LConn1
  bb -/RConn1 -- Series RLC Branch1/RConn1 -- Series RLC Branch2/RConn1 -- 2/RConn1 -- vv_2 -/RConn1
  1/RConn1 -- Series RLC Branch/LConn1 -- 2/LConn1
  Series RLC Branch/RConn1 -- vv_1 +/RConn1
  bb +/RConn1 -- Ideal Switch/LConn1

== system IOT_Charger/Subsystem3 ==
  1 : spsMosfetLib/Mosfet  Ron=0.1  Lon=0  Rd=0.01  Vfd=0  IC=0  Rs=1e5  Cs=inf  Measurements=off
  2 : spsMosfetLib/Mosfet  Ron=0.1  Lon=0  Rd=0.01  Vfd=0  IC=0  Rs=1e5  Cs=inf  Measurements=off
  Control : Subsystem
  Display : Display
  Series RLC Branch : spsSeriesRLCBranchLib/Series RLC Branch  LConnTagsString=__new0  RConnTagsString=__new0  BranchType=RL  Resistance=0.05  Inductance=5.76e-3  SetiL0=off  InitialCurrent=0  Capacitance=1e-6  Setx0=off  InitialVoltage=0  Measurements=None
  Series RLC Branch1 : spsSeriesRLCBranchLib/Series RLC Branch  LConnTagsString=__new0  RConnTagsString=__new0  BranchType=R  Resistance=5  Inductance=5.76e-4  SetiL0=off  InitialCurrent=0  Capacitance=1e-6  Setx0=off  InitialVoltage=0  Measurements=None
  Series RLC Branch2 : spsSeriesRLCBranchLib/Series RLC Branch  LConnTagsString=__new0  RConnTagsString=__new0  BranchType=RC  Resistance=0.001  Inductance=5.76e-4  SetiL0=off  InitialCurrent=0  Capacitance=1000e-6  Setx0=off  InitialVoltage=0  Measurements=None
  Voltage Measurement : spsVoltageMeasurementLib/Voltage Measurement  PhasorSimulation=off  OutputType=Complex  PSBequivalent=0
  bb - : PMIOPort  Side=Left
  bb + : PMIOPort  Port=2  Side=Left
  vv_1 + : PMIOPort  Port=3  Side=Right
  vv_2 - : PMIOPort  Port=4  Side=Right
  wires:
  [Mosfet_44] -> 1/1
  [Mosfet_444] -> 2/1
  Voltage Measurement/1 -> Display/1
  connections:
  Series RLC Branch2/LConn1 -- Series RLC Branch1/LConn1 -- bb +/RConn1 -- 1/LConn1
  bb -/RConn1 -- Series RLC Branch1/RConn1 -- Series RLC Branch2/RConn1 -- 2/RConn1 -- Voltage Measurement/LConn2 -- vv_2 -/RConn1
  1/RConn1 -- Series RLC Branch/LConn1 -- 2/LConn1
  Series RLC Branch/RConn1 -- Voltage Measurement/LConn1 -- vv_1 +/RConn1

== system IOT_Charger/Subsystem4 ==
  Constant : Constant  Value=300
  Current Measurement : spsCurrentMeasurementLib/Current Measurement  PhasorSimulation=off  OutputType=Complex  PSBequivalent=0
  Display : Display
  Display1 : Display
  Series RLC Branch : spsSeriesRLCBranchLib/Series RLC Branch  LConnTagsString=__new0  RConnTagsString=__new0  BranchType=R  Resistance=5  Inductance=1e-3  SetiL0=off  InitialCurrent=0  Capacitance=1e-6  Setx0=off  InitialVoltage=0  Measurements=None
  Subsystem : Subsystem
  Voltage Measurement : spsVoltageMeasurementLib/Voltage Measurement  PhasorSimulation=off  OutputType=Complex  PSBequivalent=0
  car + : PMIOPort  Side=Left
  car - : PMIOPort  Port=2  Side=Left
  tag scope: current_4=global, temperature_4=global, voltage_4=global
  wires:
  Current Measurement/1 -> [current_4], Display1/1
  Voltage Measurement/1 -> [voltage_4], Display/1
  Constant/1 -> [temperature_4]
  connections:
  Series RLC Branch/RConn1 -- Subsystem/LConn2 -- car -/RConn1 -- Voltage Measurement/LConn2
  Series RLC Branch/LConn1 -- Current Measurement/RConn1 -- Voltage Measurement/LConn1
  Current Measurement/LConn1 -- Subsystem/LConn1 -- car +/RConn1

== system IOT_Charger/Subsystem5 ==
  Constant : Constant  Value=300
  Display : Display
  Subsystem : Subsystem
  Voltage Measurement : spsVoltageMeasurementLib/Voltage Measurement  PhasorSimulation=off  OutputType=Complex  PSBequivalent=0
  car + : PMIOPort  Side=Left
  car - : PMIOPort  Port=2  Side=Left
  tag scope: temperature_1=global, voltage_1=global
  wires:
  Voltage Measurement/1 -> [voltage_1], Display/1
  Constant/1 -> [temperature_1]
  connections:
  Subsystem/LConn2 -- Voltage Measurement/LConn2 -- car -/RConn1
  Subsystem/LConn1 -- Voltage Measurement/LConn1 -- car +/RConn1

== system IOT_Charger/Subsystem6 ==
  Constant : Constant  Value=300
  Current Measurement : spsCurrentMeasurementLib/Current Measurement  PhasorSimulation=off  OutputType=Complex  PSBequivalent=0
  Display : Display
  Display1 : Display
  Series RLC Branch : spsSeriesRLCBranchLib/Series RLC Branch  LConnTagsString=__new0  RConnTagsString=__new0  BranchType=R  Resistance=5  Inductance=1e-3  SetiL0=off  InitialCurrent=0  Capacitance=1e-6  Setx0=off  InitialVoltage=0  Measurements=None
  Subsystem : Subsystem
  Voltage Measurement : spsVoltageMeasurementLib/Voltage Measurement  PhasorSimulation=off  OutputType=Complex  PSBequivalent=0
  car + : PMIOPort  Side=Left
  car - : PMIOPort  Port=2  Side=Left
  tag scope: current_2=global, temperature_2=global, voltage_2=global
  wires:
  Current Measurement/1 -> [current_2], Display1/1
  Voltage Measurement/1 -> [voltage_2], Display/1
  Constant/1 -> [temperature_2]
  connections:
  Series RLC Branch/RConn1 -- Subsystem/LConn2 -- car -/RConn1 -- Voltage Measurement/LConn2
  Series RLC Branch/LConn1 -- Current Measurement/RConn1 -- Voltage Measurement/LConn1
  Current Measurement/LConn1 -- Subsystem/LConn1 -- car +/RConn1

== system IOT_Charger/Subsystem7 ==
  Constant : Constant  Value=300
  Current Measurement : spsCurrentMeasurementLib/Current Measurement  PhasorSimulation=off  OutputType=Complex  PSBequivalent=0
  Display : Display
  Display1 : Display
  Series RLC Branch : spsSeriesRLCBranchLib/Series RLC Branch  LConnTagsString=__new0  RConnTagsString=__new0  BranchType=R  Resistance=5  Inductance=1e-3  SetiL0=off  InitialCurrent=0  Capacitance=1e-6  Setx0=off  InitialVoltage=0  Measurements=None
  Subsystem : Subsystem
  Voltage Measurement : spsVoltageMeasurementLib/Voltage Measurement  PhasorSimulation=off  OutputType=Complex  PSBequivalent=0
  car + : PMIOPort  Side=Left
  car - : PMIOPort  Port=2  Side=Left
  tag scope: current_3=global, temperature_3=global, voltage_3=global
  wires:
  Current Measurement/1 -> [current_3], Display1/1
  Voltage Measurement/1 -> [voltage_3], Display/1
  Constant/1 -> [temperature_3]
  connections:
  Series RLC Branch/RConn1 -- Subsystem/LConn2 -- car -/RConn1 -- Voltage Measurement/LConn2
  Series RLC Branch/LConn1 -- Current Measurement/RConn1 -- Voltage Measurement/LConn1
  Current Measurement/LConn1 -- Subsystem/LConn1 -- car +/RConn1

== system IOT_Charger/Vechicle BMS Monitoring ==
  BMS Discharge : Subsystem
  Saturation : Saturate  UpperLimit=+inf  LowerLimit=0
  wires:
  Saturation/1 -> BMS Discharge/3(Current)
  [current_4] -> Saturation/1
  [terminalvoltage_4] -> BMS Discharge/1(Terminal voltage)
  [temperature_4] -> BMS Discharge/2(Temperature)

== system IOT_Charger/Vechicle BMS Monitoring1 ==
  BMS Discharge : Subsystem
  Saturation : Saturate  UpperLimit=+inf  LowerLimit=0
  wires:
  Saturation/1 -> BMS Discharge/3(Current)
  [current_1] -> Saturation/1
  [terminalvoltage_1] -> BMS Discharge/1(Terminal voltage)
  [temperature_1] -> BMS Discharge/2(Temperature)

== system IOT_Charger/Vechicle BMS Monitoring2 ==
  BMS Discharge : Subsystem
  Saturation : Saturate  UpperLimit=+inf  LowerLimit=0
  wires:
  Saturation/1 -> BMS Discharge/3(Current)
  [current_1] -> Saturation/1
  [terminalvoltage_1] -> BMS Discharge/1(Terminal voltage)
  [temperature_1] -> BMS Discharge/2(Temperature)

== system IOT_Charger/Vechicle BMS Monitoring3 ==
  BMS Discharge : Subsystem
  Saturation : Saturate  UpperLimit=+inf  LowerLimit=0
  wires:
  Saturation/1 -> BMS Discharge/3(Current)
  [current_3] -> Saturation/1
  [terminalvoltage_3] -> BMS Discharge/1(Terminal voltage)
  [temperature_3] -> BMS Discharge/2(Temperature)

== system IOT_Charger/DC//DC converter/DC - DC Converter ==
  C : spsSeriesRLCBranchLib/Series RLC Branch  LConnTagsString=__new0  RConnTagsString=__new0  BranchType=C  Resistance=0.01  Inductance=1e-3  SetiL0=off  InitialCurrent=0  Capacitance=1000e-6  Setx0=on  InitialVoltage=200  Measurements=None
  Diode : spsDiodeLib/Diode  Ron=0.001  Lon=0  Vf=1.1  IC=0  UseSnubber=off  Rs=500  Cs=250e-9  Measurements=off
  Diode2 : spsDiodeLib/Diode  Ron=0.001  Lon=0  Vf=0.7  IC=0  UseSnubber=off  Rs=500  Cs=250e-9  Measurements=off
  IGBT : spsIGBTLib/IGBT  Ron=0.001  Lon=0  Vf=1.1  Tf=1e-6  Tt=2e-6  IC=0  Rs=1e5  Cs=inf  Measurements=off
  RL : spsSeriesRLCBranchLib/Series RLC Branch  LConnTagsString=__new0  RConnTagsString=__new0  BranchType=RL  Resistance=0.05  Inductance=470e-6  SetiL0=off  InitialCurrent=0  Capacitance=1e-6  Setx0=off  InitialVoltage=0  Measurements=None
  DC + : PMIOPort  Side=Right
  solar panel + : PMIOPort  Port=2  Side=Left
  solar panel - : PMIOPort  Port=3  Side=Left
  DC - : PMIOPort  Port=4  Side=Right
  wires:
  [Pulse_PV] -> IGBT/1
  connections:
  Diode/RConn1 -- DC +/RConn1
  Diode2/RConn1 -- C/LConn1 -- RL/LConn1
  Diode/LConn1 -- RL/RConn1 -- IGBT/LConn1
  solar panel +/RConn1 -- Diode2/LConn1
  C/RConn1 -- solar panel -/RConn1 -- DC -/RConn1 -- IGBT/RConn1

== system IOT_Charger/DC//DC converter/DC bus ==
  1 ohm 2000uH : spsSeriesRLCBranchLib/Series RLC Branch  LConnTagsString=__new0  RConnTagsString=__new0  BranchType=RC  Resistance=1  Inductance=0  SetiL0=off  InitialCurrent=0  Capacitance=2000e-6  Setx0=on  InitialVoltage=370  Measurements=None
  RL + : spsSeriesRLCBranchLib/Series RLC Branch  LConnTagsString=__new0  RConnTagsString=__new0  BranchType=RL  Resistance=0.05  Inductance=470e-6  SetiL0=off  InitialCurrent=0  Capacitance=1e-6  Setx0=off  InitialVoltage=0  Measurements=None
  RL - : spsSeriesRLCBranchLib/Series RLC Branch  LConnTagsString=__new0  RConnTagsString=__new0  BranchType=RL  Resistance=0.05  Inductance=470e-6  SetiL0=off  InitialCurrent=0  Capacitance=1e-6  Setx0=off  InitialVoltage=0  Measurements=None
  Transfer Fcn : TransferFcn  Denominator=[1e-4 1]
  V : spsVoltageMeasurementLib/Voltage Measurement  PhasorSimulation=off  OutputType=Complex  PSBequivalent=0
  left + : PMIOPort  Side=Left
  left - : PMIOPort  Port=2  Side=Left
  right + : PMIOPort  Port=3  Side=Right
  right - : PMIOPort  Port=4  Side=Right
  tag scope: Vdc=global
  wires:
  V/1 -> Transfer Fcn/1
  Transfer Fcn/1 -> [Vdc]
  connections:
  RL +/RConn1 -- 1 ohm 2000uH/LConn1 -- right +/RConn1 -- V/LConn1
  RL -/RConn1 -- 1 ohm 2000uH/RConn1 -- right -/RConn1 -- V/LConn2
  left +/RConn1 -- RL +/LConn1
  left -/RConn1 -- RL -/LConn1

== system IOT_Charger/Fast charging controller/Fast charging Switching controller ==
  g1 : Subsystem
  g2 : Subsystem
  g3 : Subsystem
  g4 : Subsystem
